simulink model "Charge_complete_V3"  (R2020a)
settings: Solver=VariableStepAuto  StartTime=0.0  StopTime=7500  RelTol=1e-3
undefined symbols (not defined in the file): Ion, Lithium
libraries: powerlib x9, electricdrivelib x1
settings Model: Creator=guill  LastModifiedBy=guill

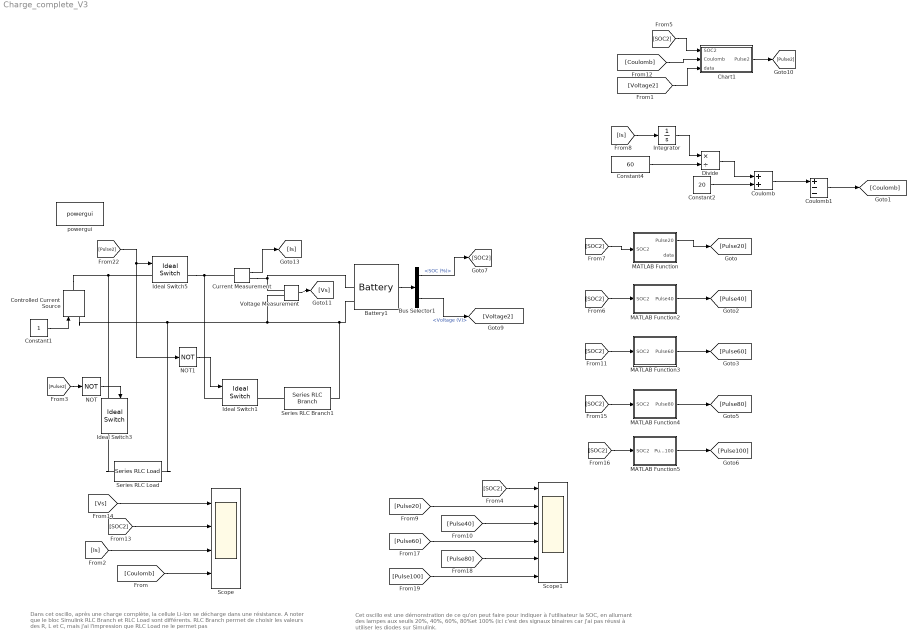
== system Charge_complete_V3 ==
  note: Dans cet oscillo, après une charge complète, la cellule Li-ion se décharge dans une résistance. A noter que le bloc Simulink RLC Branch et RLC Load sont différents. RLC Branch permet de choisir les valeurs des R, L et C, mais j'ai l'impression que RLC Load ne le permet pas
  note: Cet oscillo est une démonstration de ce qu'on peut faire pour indiquer à l'utilisateur la SOC, en allumant des lampes aux seuils 20%, 40%, 60%, 80%et 100% (ici c'est des signaux binaires car j'ai pas réussi à utiliser les diodes sur Simulink.
  Battery1 : electricdrivelib/Extra Sources/Battery  BatType=Lithium-Ion  ShowTempParam=on  ThermalPreset="3.6V  2.0Ah"  ShowAgeParam=off  NomV=3.5  NomQ=2  SOC=35  Batt_Tr=30  PresetModel=off  MaxQ=2.05  MinV=2.625  FullV=4.1  Dis_rate=0.4  R=0.017  Normal_OP=1.8087  expZone="[3.88         0.2]"  current=[6.5 13 32.5]  Units=Time  Tci=20  NomT=115  T2=0  MaxQ2=1.65  FullV2=4  Normal_OP2=3.25  expZone2="[3.8         0.2]"  Rca=0.06  ti=1000  Dp=0  Neq0=0  Tsim=1e6  Ta1=25  Qeol=5.4*0.9  Reol=0.013333*1.2  Char_age=[2.3478, 3]  Dis_age=[2.3478, 10]  N1=1500  N2=10500  N3=1000  N4=1400  Ta2=45  N5=950
  Bus Selector1 : BusSelector  OutputSignals=SOC (%),Current (A),Voltage (V)
  Chart1 : Stateflow chart  TreatAsAtomicUnit=on
  Constant1 : Constant
  Constant2 : Constant  Value=20
  Constant4 : Constant  Value=60
  Controlled Current Source : powerlib/Electrical Sources/Controlled Current Source  Initialize=on  Source_Type=AC  Amplitude=0  Phase=0  Frequency=0  Measurements=None
  Coulomb : Sum
  Coulomb1 : Sum  Inputs=+--
  Current Measurement : powerlib/Measurements/Current Measurement  PhasorSimulation=off  OutputType=Complex  PSBequivalent=0
  Divide : Product  Inputs=*/
  Ideal Switch1 : powerlib/Power Electronics/Ideal Switch  Ron=0.001  Lon=0  IC=0  Rs=1e5  Cs=inf  Measurements=on
  Ideal Switch3 : powerlib/Power Electronics/Ideal Switch  Ron=0.001  Lon=0  IC=0  Rs=1e5  Cs=inf  Measurements=on
  Ideal Switch5 : powerlib/Power Electronics/Ideal Switch  Ron=0.001  Lon=0  IC=0  Rs=1e5  Cs=inf  Measurements=on
  Integrator : Integrator
  MATLAB Function : MATLAB Function  TreatAsAtomicUnit=on
  MATLAB Function2 : MATLAB Function  TreatAsAtomicUnit=on
  MATLAB Function3 : MATLAB Function  TreatAsAtomicUnit=on
  MATLAB Function4 : MATLAB Function  TreatAsAtomicUnit=on
  MATLAB Function5 : MATLAB Function  TreatAsAtomicUnit=on
  NOT : Logic  Operator=NOT  IconShape=distinctive  AllPortsSameDT=off  OutDataTypeStr=boolean
  NOT1 : Logic  Operator=NOT  IconShape=distinctive  AllPortsSameDT=off  OutDataTypeStr=boolean
  Scope : Scope  NumInputPorts=4
  Scope1 : Scope  NumInputPorts=6
  Series RLC Branch1 : powerlib/Elements/Series RLC Branch  LConnTagsString=__new0  RConnTagsString=__new0  BranchType=RLC  Resistance=1  Inductance=0  SetiL0=off  InitialCurrent=0  Capacitance=0  Setx0=off  InitialVoltage=0  Measurements=None
  Series RLC Load : powerlib/Elements/Series RLC Load  LConnTagsString=a  RConnTagsString=__new0  NominalVoltage=10  NominalFrequency=60  ActivePower=1000  InductivePower=0  CapacitivePower=0  Setx0=off  InitialVoltage=0  SetiL0=off  InitialCurrent=0  Measurements=None  LoadType=constant Z
  Voltage Measurement : powerlib/Measurements/Voltage Measurement  PhasorSimulation=off  OutputType=Complex  PSBequivalent=0
  powergui : powerlib/powergui  Priority=1  SimulationMode=Continuous  SampleTime=50e-2  frequency=60  Iterations=50  frequencyindice=0  Pbase=100e6  ErrMax=1e-4  UnitsV=kV  UnitsW=MW  buscounter=0  FunctionMessages=off  echomessages=off  EnableUseOfTLC=off  CurrentSourceSwitches=off  DisableSnubberDevices=off  DisableRonSwitches=off  DisableVfSwitches=off  DisplayEquations=off  AutomaticDiscreteSolvers=off  SolverType=Tustin/Backward Euler (TBE)  Interpol=off  ExternalGateDelay=off  methode=off  Ts=100  x0status=blocks  SPID=on  SwTol=0  HookPort=off  NonlinearTolerance=1e-4  nMaxIteration=100  ContinueOnMaxIteration=off  RestoreLinks=warning  ResistiveCurrentMeasurement=off  Frange=[0:2:500]  Ylog=off  Xlog=on  ShowGrid=off  save=off  variable=ZData  structure=0  ZoomFFT=off  StartTime=0.0  cycles=1  DisplayStyle=1  fundamental=60  FreqAxis=off  MaxFrequency=1000  frequencyindicesteady=1  RmsSteady=1  display=off
  wires:
  [Is] -> Scope/3
  Coulomb/1 -> Coulomb1/1
  Constant2/1 -> Coulomb/2
  [Pulse2] -> NOT1/1, Ideal Switch5/1
  Bus Selector1/1 -> [SOC2]  "<SOC (%)>"
  Integrator/1 -> Divide/1
  Divide/1 -> Coulomb/1
  [SOC2] -> Scope/2
  Constant1/1 -> Controlled Current Source/1
  NOT/1 -> Ideal Switch3/1
  Battery1/1 -> Bus Selector1/1
  Current Measurement/1 -> [Is]
  Bus Selector1/3 -> [Voltage2]  "<Voltage (V)>"
  [Pulse2] -> NOT/1
  [Coulomb] -> Scope/4
  Constant4/1 -> Divide/2
  [Vs] -> Scope/1
  Voltage Measurement/1 -> [Vs]
  [Coulomb] -> Chart1/2(Coulomb)
  [Is] -> Integrator/1
  [Voltage2] -> Chart1/3(data)
  [SOC2] -> Chart1/1(SOC2)
  Chart1/1(Pulse2) -> [Pulse2]
  Coulomb1/1 -> [Coulomb]
  NOT1/1 -> Ideal Switch1/1
  MATLAB Function/1(Pulse20) -> [Pulse20]
  MATLAB Function3/1(Pulse60) -> [Pulse60]
  [SOC2] -> MATLAB Function4/1(SOC2)
  [SOC2] -> MATLAB Function3/1(SOC2)
  MATLAB Function2/1(Pulse40) -> [Pulse40]
  [SOC2] -> MATLAB Function/1(SOC2)
  MATLAB Function5/1(Pulse100) -> [Pulse100]
  [SOC2] -> MATLAB Function2/1(SOC2)
  [SOC2] -> MATLAB Function5/1(SOC2)
  MATLAB Function4/1(Pulse80) -> [Pulse80]
  [SOC2] -> Scope1/1
  [Pulse20] -> Scope1/2
  [Pulse40] -> Scope1/3
  [Pulse60] -> Scope1/4
  [Pulse80] -> Scope1/5
  [Pulse100] -> Scope1/6
  connections:
  Controlled Current Source/RConn1 -- Ideal Switch5/LConn1 -- Ideal Switch3/LConn1
  Controlled Current Source/LConn1 -- Series RLC Branch1/RConn1 -- Battery1/LConn2 -- Voltage Measurement/LConn2 -- Series RLC Load/RConn1
  Current Measurement/RConn1 -- Battery1/LConn1 -- Voltage Measurement/LConn1
  Series RLC Load/LConn1 -- Ideal Switch3/RConn1
  Ideal Switch5/RConn1 -- Ideal Switch1/LConn1 -- Current Measurement/LConn1
  Series RLC Branch1/LConn1 -- Ideal Switch1/RConn1

== stateflow chart Charge_complete_V3/Chart1 ==
  state Charge2
    entry: Pulse2=1
  state Discharge2
    entry: Pulse2=0
  (default) -> Charge2
  Charge2 -> Discharge2 : [Coulomb>98]
  Discharge2 -> Charge2 : [Coulomb<20]
  data: SOC2 input; Pulse2 output; Coulomb input; data input

== matlab function Charge_complete_V3/MATLAB Function2 ==
  data: SOC2 input; Pulse40 output
function Pulse40 = fcn(SOC2)
if SOC2>40
    Pulse40=1;
else
    Pulse40=0;
end
end

== matlab function Charge_complete_V3/MATLAB Function ==
  data: SOC2 input; Pulse20 output; data output
function [Pulse20,data] = fcn(SOC2)
if SOC2>20
    Pulse20=1;
else
    Pulse20=0;
end
end

== matlab function Charge_complete_V3/MATLAB Function3 ==
  data: SOC2 input; Pulse60 output
function Pulse60 = fcn(SOC2)
if SOC2>60
    Pulse60=1;
else
    Pulse60=0;
end
end

== matlab function Charge_complete_V3/MATLAB Function4 ==
  data: SOC2 input; Pulse80 output
function Pulse80 = fcn(SOC2)
if SOC2>80
    Pulse80=1;
else
    Pulse80=0;
end
end

== matlab function Charge_complete_V3/MATLAB Function5 ==
  data: SOC2 input; Pulse100 output
function Pulse100 = fcn(SOC2)
if SOC2>100
    Pulse100=1;
else
    Pulse100=0;
end
end
